simulink subsystem "MFTiresMultibodyFrontSSC"  (R2024a)
settings: Solver=VariableStepAuto  StartTime=0.0  StopTime=10.0  RelTol=1e-3
undefined symbols (not defined in the file): Alpha, AxlFL, AxlFR, AxlTrq, BrkPrs, Fx, Fy, Fz, Gamma, Kappa, Mx, My, Mz, Omega, PlntVehMultiBody, psidot, Re, Vx, Vy, WheelFL, WheelFR, X, Y, Z
libraries: nesl_utility x34, sm_lib x34, fl_lib x6
(part 2 of 2)

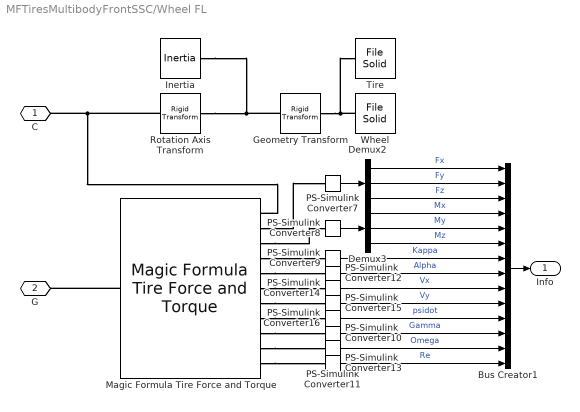
== system MFTiresMultibodyFrontSSC/Wheel FL ==
  Bus Creator1 : BusCreator  Inputs=14
  Demux2 : Demux  Outputs=3
  Demux3 : Demux  Outputs=3
  Geometry Transform : sm_lib/Frames and Transforms/Rigid Transform  RotationMethod=StandardAxis  FollAlignAxisA=+X  BaseAlignAxisA=+Y  FollAlignAxisB=+Y  BaseAlignAxisB=+Z  RotationStandardAxis=+X  RotationAngle=sideSign*180-90  RotationAngleUnits=deg  RotationArbitraryAxis=[0 0 1]  RotationSequenceAxes=FollowerAxes  RotationSequence=XYX  RotationSequenceAngles=[0 0 0]  RotationSequenceAnglesUnits=deg  RotationMatrix=[1 0 0; 0 1 0; 0 0 1]  Quaternion=[1 0 0 0]  TranslationMethod=StandardAxis  TranslationCartesianOffset=[0 0 0]  TranslationCartesianOffsetUnits=m  TranslationStandardAxis=+Y  TranslationStandardOffset=(1-2*sideSign)*0.125  TranslationStandardOffsetUnits=m  TranslationROffset=0  TranslationROffsetUnits=m  TranslationThetaOffset=0  TranslationThetaOffsetUnits=deg  TranslationZOffset=0  TranslationZOffsetUnits=m
  Inertia : sm_lib/Body Elements/Inertia  InertiaType=Custom  Mass=wheelAssm_mass  MassUnits=kg  CenterOfMass=[0 0 0]  CenterOfMassUnits=m  MomentsOfInertia=wheelAssm_I  MomentsOfInertiaUnits=kg*m^2  ProductsOfInertia=[0 0 0]  ProductsOfInertiaUnits=kg*m^2  GraphicType=None  MarkerShape=Inertia  MarkerSize=20  GraphicVisPropType=SimpleVisualProperties  GraphicDiffuseColor=[0.5 0.5 0.5]  GraphicOpacity=1.0  GraphicSpecularColor=[0.5 0.5 0.5 1.0]  GraphicAmbientColor=[0.15 0.15 0.15 1.0]  GraphicEmissiveColor=[0.0 0.0 0.0 1.0]  GraphicShininess=75
  Magic Formula Tire Force and Torque : sm_lib/Forces and Torques/Magic Formula Tire Force and Torque  TireSide=Left  TireParameters=tire_param  SlipMode=Combined  ScalingCoefficientLMUXMode=FromTireParameters  ScalingCoefficientLMUYMode=FromTireParameters  SenseContactSignal=off  TireWrenchFrame=ContactFrame  SenseTireForce=on  SenseTireTorque=on  SensePneumaticTrail=off  SenseLongitudinalSlip=on  SenseSaturatedLongitudinalSlip=off  SenseSlipAngle=on  SenseSaturatedSlipAngle=off  SenseTurnSlip=off  SenseRelativeLongitudinalVelocity=on  SenseRelativeLateralVelocity=on  SenseLongitudinalSlipVelocity=off  SenseLateralSlipVelocity=off  SenseYawVelocity=on  SenseCamberAngle=on  SenseSaturatedCamberAngle=off  SenseCamberVelocity=off  SenseSpinVelocity=on  SenseFreeRadius=off  SenseLoadedRadius=off  SenseEffectiveRollingRadius=on  SenseLongitudinalFrictionCoefficient=off  SenseLateralFrictionCoefficient=off  SenseContactBaseRotation=off  SenseContactBaseTranslation=off  SenseContactFollowerRotation=off  SenseContactFollowerTranslation=off  NumericParameters=[0.1 0.1 0.1 0.1 0.1 1e-4 1e-4 1e-7 1e-7 1e-4 1e-4 0.1 1e-4 1e-4 1e-4 1e-4 1e-4 1e-4 1e-4 1e-4 1e-4]
  PS-Simulink Converter{7..16} (10 alike) : nesl_utility/PS-Simulink Converter  PhysicalDomain=network_engine_domain  SubClassName=ps_output  LeftPortType=input  RightPortType=output  PseudoPeriodic=off  Frequencies=[]  VectorFormat=1-D array  Unit=inherit  AffineConversion=off
  Rotation Axis Transform : sm_lib/Frames and Transforms/Rigid Transform  RotationMethod=AlignedAxes  FollAlignAxisA=+X  BaseAlignAxisA=+X  FollAlignAxisB=+Z  BaseAlignAxisB=+Y  RotationStandardAxis=-X  RotationAngle=0  RotationAngleUnits=deg  RotationArbitraryAxis=[0 0 1]  RotationSequenceAxes=FollowerAxes  RotationSequence=XYX  RotationSequenceAngles=[0 0 0]  RotationSequenceAnglesUnits=deg  RotationMatrix=[1 0 0; 0 1 0; 0 0 1]  Quaternion=[1 0 0 0]  TranslationMethod=None  TranslationCartesianOffset=[0 0 0]  TranslationCartesianOffsetUnits=m  TranslationStandardAxis=+Z  TranslationStandardOffset=0  TranslationStandardOffsetUnits=m  TranslationROffset=0  TranslationROffsetUnits=m  TranslationThetaOffset=0  TranslationThetaOffsetUnits=deg  TranslationZOffset=0  TranslationZOffsetUnits=m
  Tire : sm_lib/Body Elements/File Solid  ExtGeomFileName=sm_car_heave_roll_tire.STL  UnitType=Custom  ExtGeomFileUnits=mm  StepReaderType=HEX  ExportConvexHullGeometry=off  InertiaType=Custom  BasedOnType=Density  Density=1000  DensityUnits=kg/m^3  Mass=0  MassUnits=kg  CenterOfMass=[0 0 0]  CenterOfMassUnits=m  MomentsOfInertia=[0 0 0]  MomentsOfInertiaUnits=kg*m^2  ProductsOfInertia=[0 0 0]  ProductsOfInertiaUnits=kg*m^2  GraphicType=FromGeometry  MarkerShape=Sphere  MarkerSize=10  GraphicVisPropType=SimpleVisualProperties  GraphicDiffuseColor=[0.5 0.5 0.5]  GraphicOpacity=1.0  GraphicSpecularColor=[0.5 0.5 0.5 1.0]  GraphicAmbientColor=[0.15 0.15 0.15 1.0]  GraphicEmissiveColor=[0.0 0.0 0.0 1.0]  GraphicShininess=75  DoExposeReferenceFrame=on  SerializedFrames=<Frames/>
  Wheel : sm_lib/Body Elements/File Solid  ExtGeomFileName=sm_car_heave_roll_wheel.STL  UnitType=Custom  ExtGeomFileUnits=mm  StepReaderType=HEX  ExportConvexHullGeometry=off  InertiaType=Custom  BasedOnType=Density  Density=1000  DensityUnits=kg/m^3  Mass=0  MassUnits=kg  CenterOfMass=[0 0 0]  CenterOfMassUnits=m  MomentsOfInertia=[0 0 0]  MomentsOfInertiaUnits=kg*m^2  ProductsOfInertia=[0 0 0]  ProductsOfInertiaUnits=kg*m^2  GraphicType=FromGeometry  MarkerShape=Sphere  MarkerSize=10  GraphicVisPropType=SimpleVisualProperties  GraphicDiffuseColor=[0.8 0.8 0.8]  GraphicOpacity=1.0  GraphicSpecularColor=[0.5 0.5 0.5 1.0]  GraphicAmbientColor=[0.15 0.15 0.15 1.0]  GraphicEmissiveColor=[0.0 0.0 0.0 1.0]  GraphicShininess=75  DoExposeReferenceFrame=on  SerializedFrames=<Frames/>
  C : PMIOPort  Side=Left
  G : PMIOPort  Port=2  Side=Right
  Info : Outport
  wires:
  Bus Creator1/1 -> Info/1
  Demux3/1 -> Bus Creator1/4  "Mx"
  PS-Simulink Converter12/1 -> Bus Creator1/8  "Alpha"
  PS-Simulink Converter10/1 -> Bus Creator1/12  "Gamma"
  Demux3/2 -> Bus Creator1/5  "My"
  PS-Simulink Converter8/1 -> Demux3/1
  Demux3/3 -> Bus Creator1/6  "Mz"
  Demux2/3 -> Bus Creator1/3  "Fz"
  PS-Simulink Converter16/1 -> Bus Creator1/11  "psidot"
  PS-Simulink Converter9/1 -> Bus Creator1/7  "Kappa"
  Demux2/2 -> Bus Creator1/2  "Fy"
  PS-Simulink Converter11/1 -> Bus Creator1/13  "Omega"
  PS-Simulink Converter15/1 -> Bus Creator1/10  "Vy"
  PS-Simulink Converter7/1 -> Demux2/1
  Demux2/1 -> Bus Creator1/1  "Fx"
  PS-Simulink Converter14/1 -> Bus Creator1/9  "Vx"
  PS-Simulink Converter13/1 -> Bus Creator1/14  "Re"
  connections:
  Magic Formula Tire Force and Torque/RConn3 -- PS-Simulink Converter8/LConn1
  Magic Formula Tire Force and Torque/RConn11 -- PS-Simulink Converter13/LConn1
  Magic Formula Tire Force and Torque/RConn7 -- PS-Simulink Converter15/LConn1
  Magic Formula Tire Force and Torque/RConn4 -- PS-Simulink Converter9/LConn1
  Magic Formula Tire Force and Torque/LConn1 -- G/RConn1
  Magic Formula Tire Force and Torque/RConn10 -- PS-Simulink Converter11/LConn1
  Magic Formula Tire Force and Torque/RConn8 -- PS-Simulink Converter16/LConn1
  Magic Formula Tire Force and Torque/RConn2 -- PS-Simulink Converter7/LConn1
  Magic Formula Tire Force and Torque/RConn5 -- PS-Simulink Converter12/LConn1
  Magic Formula Tire Force and Torque/RConn6 -- PS-Simulink Converter14/LConn1
  Magic Formula Tire Force and Torque/RConn9 -- PS-Simulink Converter10/LConn1
  Wheel/RConn1 -- Geometry Transform/RConn1 -- Tire/RConn1
  Inertia/RConn1 -- Geometry Transform/LConn1 -- Rotation Axis Transform/LConn1
  Magic Formula Tire Force and Torque/RConn1 -- Rotation Axis Transform/RConn1 -- C/RConn1

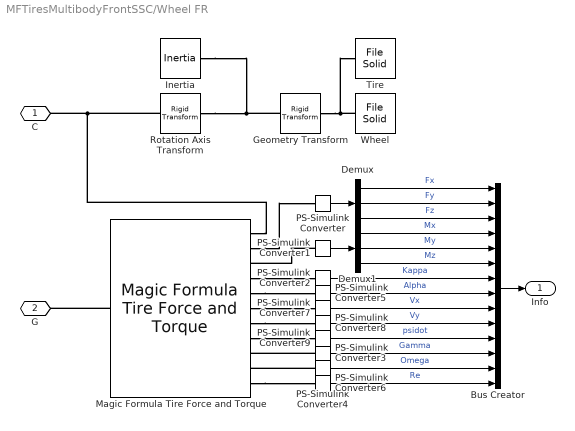
== system MFTiresMultibodyFrontSSC/Wheel FR ==
  Bus Creator : BusCreator  Inputs=14
  Demux : Demux  Outputs=3
  Demux1 : Demux  Outputs=3
  Geometry Transform : sm_lib/Frames and Transforms/Rigid Transform  RotationMethod=StandardAxis  FollAlignAxisA=+X  BaseAlignAxisA=+Y  FollAlignAxisB=+Y  BaseAlignAxisB=+Z  RotationStandardAxis=+X  RotationAngle=sideSign*180-90  RotationAngleUnits=deg  RotationArbitraryAxis=[0 0 1]  RotationSequenceAxes=FollowerAxes  RotationSequence=XYX  RotationSequenceAngles=[0 0 0]  RotationSequenceAnglesUnits=deg  RotationMatrix=[1 0 0; 0 1 0; 0 0 1]  Quaternion=[1 0 0 0]  TranslationMethod=StandardAxis  TranslationCartesianOffset=[0 0 0]  TranslationCartesianOffsetUnits=m  TranslationStandardAxis=+Y  TranslationStandardOffset=(1-2*sideSign)*0.125  TranslationStandardOffsetUnits=m  TranslationROffset=0  TranslationROffsetUnits=m  TranslationThetaOffset=0  TranslationThetaOffsetUnits=deg  TranslationZOffset=0  TranslationZOffsetUnits=m
  Inertia : sm_lib/Body Elements/Inertia  InertiaType=Custom  Mass=wheelAssm_mass  MassUnits=kg  CenterOfMass=[0 0 0]  CenterOfMassUnits=m  MomentsOfInertia=wheelAssm_I  MomentsOfInertiaUnits=kg*m^2  ProductsOfInertia=[0 0 0]  ProductsOfInertiaUnits=kg*m^2  GraphicType=None  MarkerShape=Inertia  MarkerSize=20  GraphicVisPropType=SimpleVisualProperties  GraphicDiffuseColor=[0.5 0.5 0.5]  GraphicOpacity=1.0  GraphicSpecularColor=[0.5 0.5 0.5 1.0]  GraphicAmbientColor=[0.15 0.15 0.15 1.0]  GraphicEmissiveColor=[0.0 0.0 0.0 1.0]  GraphicShininess=75
  Magic Formula Tire Force and Torque : sm_lib/Forces and Torques/Magic Formula Tire Force and Torque  TireSide=Right  TireParameters=tire_param  SlipMode=Combined  ScalingCoefficientLMUXMode=FromTireParameters  ScalingCoefficientLMUYMode=FromTireParameters  SenseContactSignal=off  TireWrenchFrame=ContactFrame  SenseTireForce=on  SenseTireTorque=on  SensePneumaticTrail=off  SenseLongitudinalSlip=on  SenseSaturatedLongitudinalSlip=off  SenseSlipAngle=on  SenseSaturatedSlipAngle=off  SenseTurnSlip=off  SenseRelativeLongitudinalVelocity=on  SenseRelativeLateralVelocity=on  SenseLongitudinalSlipVelocity=off  SenseLateralSlipVelocity=off  SenseYawVelocity=on  SenseCamberAngle=on  SenseSaturatedCamberAngle=off  SenseCamberVelocity=off  SenseSpinVelocity=on  SenseFreeRadius=off  SenseLoadedRadius=off  SenseEffectiveRollingRadius=on  SenseLongitudinalFrictionCoefficient=off  SenseLateralFrictionCoefficient=off  SenseContactBaseRotation=off  SenseContactBaseTranslation=off  SenseContactFollowerRotation=off  SenseContactFollowerTranslation=off  NumericParameters=[0.1 0.1 0.1 0.1 0.1 1e-4 1e-4 1e-7 1e-7 1e-4 1e-4 0.1 1e-4 1e-4 1e-4 1e-4 1e-4 1e-4 1e-4 1e-4 1e-4]
  PS-Simulink Converter{,1..9} (10 alike) : nesl_utility/PS-Simulink Converter  PhysicalDomain=network_engine_domain  SubClassName=ps_output  LeftPortType=input  RightPortType=output  PseudoPeriodic=off  Frequencies=[]  VectorFormat=1-D array  Unit=inherit  AffineConversion=off
  Rotation Axis Transform : sm_lib/Frames and Transforms/Rigid Transform  RotationMethod=AlignedAxes  FollAlignAxisA=+X  BaseAlignAxisA=+X  FollAlignAxisB=+Z  BaseAlignAxisB=+Y  RotationStandardAxis=-X  RotationAngle=0  RotationAngleUnits=deg  RotationArbitraryAxis=[0 0 1]  RotationSequenceAxes=FollowerAxes  RotationSequence=XYX  RotationSequenceAngles=[0 0 0]  RotationSequenceAnglesUnits=deg  RotationMatrix=[1 0 0; 0 1 0; 0 0 1]  Quaternion=[1 0 0 0]  TranslationMethod=None  TranslationCartesianOffset=[0 0 0]  TranslationCartesianOffsetUnits=m  TranslationStandardAxis=+Z  TranslationStandardOffset=0  TranslationStandardOffsetUnits=m  TranslationROffset=0  TranslationROffsetUnits=m  TranslationThetaOffset=0  TranslationThetaOffsetUnits=deg  TranslationZOffset=0  TranslationZOffsetUnits=m
  Tire : sm_lib/Body Elements/File Solid  ExtGeomFileName=sm_car_heave_roll_tire.STL  UnitType=Custom  ExtGeomFileUnits=mm  StepReaderType=HEX  ExportConvexHullGeometry=off  InertiaType=Custom  BasedOnType=Density  Density=1000  DensityUnits=kg/m^3  Mass=0  MassUnits=kg  CenterOfMass=[0 0 0]  CenterOfMassUnits=m  MomentsOfInertia=[0 0 0]  MomentsOfInertiaUnits=kg*m^2  ProductsOfInertia=[0 0 0]  ProductsOfInertiaUnits=kg*m^2  GraphicType=FromGeometry  MarkerShape=Sphere  MarkerSize=10  GraphicVisPropType=SimpleVisualProperties  GraphicDiffuseColor=[0.5 0.5 0.5]  GraphicOpacity=1.0  GraphicSpecularColor=[0.5 0.5 0.5 1.0]  GraphicAmbientColor=[0.15 0.15 0.15 1.0]  GraphicEmissiveColor=[0.0 0.0 0.0 1.0]  GraphicShininess=75  DoExposeReferenceFrame=on  SerializedFrames=<Frames/>
  Wheel : sm_lib/Body Elements/File Solid  ExtGeomFileName=sm_car_heave_roll_wheel.STL  UnitType=Custom  ExtGeomFileUnits=mm  StepReaderType=HEX  ExportConvexHullGeometry=off  InertiaType=Custom  BasedOnType=Density  Density=1000  DensityUnits=kg/m^3  Mass=0  MassUnits=kg  CenterOfMass=[0 0 0]  CenterOfMassUnits=m  MomentsOfInertia=[0 0 0]  MomentsOfInertiaUnits=kg*m^2  ProductsOfInertia=[0 0 0]  ProductsOfInertiaUnits=kg*m^2  GraphicType=FromGeometry  MarkerShape=Sphere  MarkerSize=10  GraphicVisPropType=SimpleVisualProperties  GraphicDiffuseColor=[0.8 0.8 0.8]  GraphicOpacity=1.0  GraphicSpecularColor=[0.5 0.5 0.5 1.0]  GraphicAmbientColor=[0.15 0.15 0.15 1.0]  GraphicEmissiveColor=[0.0 0.0 0.0 1.0]  GraphicShininess=75  DoExposeReferenceFrame=on  SerializedFrames=<Frames/>
  C : PMIOPort  Side=Left
  G : PMIOPort  Port=2  Side=Right
  Info : Outport
  wires:
  PS-Simulink Converter7/1 -> Bus Creator/9  "Vx"
  PS-Simulink Converter8/1 -> Bus Creator/10  "Vy"
  PS-Simulink Converter9/1 -> Bus Creator/11  "psidot"
  PS-Simulink Converter3/1 -> Bus Creator/12  "Gamma"
  PS-Simulink Converter5/1 -> Bus Creator/8  "Alpha"
  PS-Simulink Converter6/1 -> Bus Creator/14  "Re"
  PS-Simulink Converter4/1 -> Bus Creator/13  "Omega"
  PS-Simulink Converter2/1 -> Bus Creator/7  "Kappa"
  PS-Simulink Converter/1 -> Demux/1
  Demux/1 -> Bus Creator/1  "Fx"
  Demux/2 -> Bus Creator/2  "Fy"
  Demux/3 -> Bus Creator/3  "Fz"
  Demux1/3 -> Bus Creator/6  "Mz"
  Demux1/2 -> Bus Creator/5  "My"
  Demux1/1 -> Bus Creator/4  "Mx"
  PS-Simulink Converter1/1 -> Demux1/1
  Bus Creator/1 -> Info/1
  connections:
  Magic Formula Tire Force and Torque/RConn8 -- PS-Simulink Converter9/LConn1
  Magic Formula Tire Force and Torque/RConn7 -- PS-Simulink Converter8/LConn1
  Magic Formula Tire Force and Torque/RConn6 -- PS-Simulink Converter7/LConn1
  Magic Formula Tire Force and Torque/RConn11 -- PS-Simulink Converter6/LConn1
  Magic Formula Tire Force and Torque/RConn5 -- PS-Simulink Converter5/LConn1
  PS-Simulink Converter4/LConn1 -- Magic Formula Tire Force and Torque/RConn10
  PS-Simulink Converter3/LConn1 -- Magic Formula Tire Force and Torque/RConn9
  Magic Formula Tire Force and Torque/RConn4 -- PS-Simulink Converter2/LConn1
  Wheel/RConn1 -- Geometry Transform/RConn1 -- Tire/RConn1
  Inertia/RConn1 -- Geometry Transform/LConn1 -- Rotation Axis Transform/LConn1
  Magic Formula Tire Force and Torque/LConn1 -- G/RConn1
  Magic Formula Tire Force and Torque/RConn2 -- PS-Simulink Converter/LConn1
  PS-Simulink Converter1/LConn1 -- Magic Formula Tire Force and Torque/RConn3
  Rotation Axis Transform/RConn1 -- Magic Formula Tire Force and Torque/RConn1 -- C/RConn1

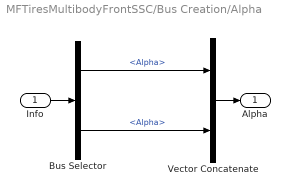
== system MFTiresMultibodyFrontSSC/Bus Creation/Alpha ==
  Info : Inport
  Bus Selector : BusSelector  OutputSignals=L.Alpha,R.Alpha
  Vector Concatenate : Concatenate
  Alpha : Outport  VectorParamsAs1DForOutWhenUnconnected=off
  wires:
  Vector Concatenate/1 -> Alpha/1
  Info/1 -> Bus Selector/1
  Bus Selector/2 -> Vector Concatenate/2  "<Alpha>"
  Bus Selector/1 -> Vector Concatenate/1  "<Alpha>"

== system MFTiresMultibodyFrontSSC/Bus Creation/BrkPrs1 ==
  In1 : Inport
  BrkPrs : Outport  VectorParamsAs1DForOutWhenUnconnected=off
  wires:
  In1/1 -> BrkPrs/1  "BrkPrs"

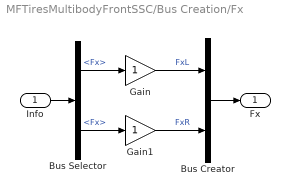
== system MFTiresMultibodyFrontSSC/Bus Creation/Fx ==
  Info : Inport
  Bus Creator : BusCreator  Inputs=2
  Bus Selector : BusSelector  OutputSignals=L.Fx,R.Fx
  Gain : Gain
  Gain1 : Gain
  Fx : Outport  VectorParamsAs1DForOutWhenUnconnected=off
  wires:
  Info/1 -> Bus Selector/1
  Bus Creator/1 -> Fx/1
  Gain1/1 -> Bus Creator/2  "FxR"
  Gain/1 -> Bus Creator/1  "FxL"
  Bus Selector/1 -> Gain/1  "<Fx>"
  Bus Selector/2 -> Gain1/1  "<Fx>"

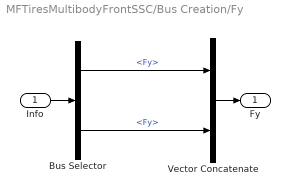
== system MFTiresMultibodyFrontSSC/Bus Creation/Fy ==
  Info : Inport
  Bus Selector : BusSelector  OutputSignals=L.Fy,R.Fy
  Vector Concatenate : Concatenate
  Fy : Outport  VectorParamsAs1DForOutWhenUnconnected=off
  wires:
  Bus Selector/2 -> Vector Concatenate/2  "<Fy>"
  Bus Selector/1 -> Vector Concatenate/1  "<Fy>"
  Vector Concatenate/1 -> Fy/1
  Info/1 -> Bus Selector/1

== system MFTiresMultibodyFrontSSC/Bus Creation/Fz ==
  Info : Inport
  Bus Selector : BusSelector  OutputSignals=L.Fz,R.Fz
  Vector Concatenate : Concatenate
  Fz : Outport  VectorParamsAs1DForOutWhenUnconnected=off
  wires:
  Bus Selector/2 -> Vector Concatenate/2  "<Fz>"
  Bus Selector/1 -> Vector Concatenate/1  "<Fz>"
  Vector Concatenate/1 -> Fz/1
  Info/1 -> Bus Selector/1

== system MFTiresMultibodyFrontSSC/Bus Creation/Gamma ==
  Info : Inport
  Bus Selector : BusSelector  OutputSignals=L.Gamma,R.Gamma
  Vector Concatenate : Concatenate
  Gamma : Outport  VectorParamsAs1DForOutWhenUnconnected=off
  wires:
  Bus Selector/1 -> Vector Concatenate/1  "<Gamma>"
  Bus Selector/2 -> Vector Concatenate/2  "<Gamma>"
  Info/1 -> Bus Selector/1
  Vector Concatenate/1 -> Gamma/1

== system MFTiresMultibodyFrontSSC/Bus Creation/Kappa ==
  Info : Inport
  Bus Selector : BusSelector  OutputSignals=L.Kappa,R.Kappa
  Vector Concatenate : Concatenate
  Kappa : Outport  VectorParamsAs1DForOutWhenUnconnected=off
  wires:
  Vector Concatenate/1 -> Kappa/1
  Info/1 -> Bus Selector/1
  Bus Selector/2 -> Vector Concatenate/2  "<Kappa>"
  Bus Selector/1 -> Vector Concatenate/1  "<Kappa>"

== system MFTiresMultibodyFrontSSC/Bus Creation/Mx ==
  Info : Inport
  Bus Selector : BusSelector  OutputSignals=L.Mx,R.Mx
  Vector Concatenate : Concatenate
  Mx : Outport  VectorParamsAs1DForOutWhenUnconnected=off
  wires:
  Bus Selector/2 -> Vector Concatenate/2  "<Mx>"
  Bus Selector/1 -> Vector Concatenate/1  "<Mx>"
  Vector Concatenate/1 -> Mx/1
  Info/1 -> Bus Selector/1

== system MFTiresMultibodyFrontSSC/Bus Creation/My ==
  Info : Inport
  Bus Selector : BusSelector  OutputSignals=L.My,R.My
  Vector Concatenate : Concatenate
  My : Outport  VectorParamsAs1DForOutWhenUnconnected=off
  wires:
  Bus Selector/2 -> Vector Concatenate/2  "<My>"
  Bus Selector/1 -> Vector Concatenate/1  "<My>"
  Vector Concatenate/1 -> My/1
  Info/1 -> Bus Selector/1

== system MFTiresMultibodyFrontSSC/Bus Creation/Mz ==
  Info : Inport
  Bus Selector : BusSelector  OutputSignals=L.Mz,R.Mz
  Vector Concatenate : Concatenate
  Mz : Outport  VectorParamsAs1DForOutWhenUnconnected=off
  wires:
  Bus Selector/2 -> Vector Concatenate/2  "<Mz>"
  Bus Selector/1 -> Vector Concatenate/1  "<Mz>"
  Vector Concatenate/1 -> Mz/1
  Info/1 -> Bus Selector/1

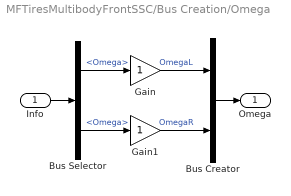
== system MFTiresMultibodyFrontSSC/Bus Creation/Omega ==
  Info : Inport
  Bus Creator : BusCreator  Inputs=2
  Bus Selector : BusSelector  OutputSignals=L.Omega,R.Omega
  Gain : Gain
  Gain1 : Gain
  Omega : Outport  VectorParamsAs1DForOutWhenUnconnected=off
  wires:
  Bus Selector/2 -> Gain1/1  "<Omega>"
  Bus Creator/1 -> Omega/1
  Info/1 -> Bus Selector/1
  Bus Selector/1 -> Gain/1  "<Omega>"
  Gain/1 -> Bus Creator/1  "OmegaL"
  Gain1/1 -> Bus Creator/2  "OmegaR"

== system MFTiresMultibodyFrontSSC/Bus Creation/Re ==
  Info : Inport
  Bus Selector : BusSelector  OutputSignals=L.Re,R.Re
  Vector Concatenate : Concatenate
  Re : Outport  VectorParamsAs1DForOutWhenUnconnected=off
  wires:
  Vector Concatenate/1 -> Re/1
  Info/1 -> Bus Selector/1
  Bus Selector/2 -> Vector Concatenate/2  "<Re>"
  Bus Selector/1 -> Vector Concatenate/1  "<Re>"

== system MFTiresMultibodyFrontSSC/Bus Creation/Vx ==
  Info : Inport
  Bus Selector : BusSelector  OutputSignals=L.Vx,R.Vx
  Vector Concatenate : Concatenate
  Vx : Outport  VectorParamsAs1DForOutWhenUnconnected=off
  wires:
  Bus Selector/1 -> Vector Concatenate/1  "<Vx>"
  Bus Selector/2 -> Vector Concatenate/2  "<Vx>"
  Info/1 -> Bus Selector/1
  Vector Concatenate/1 -> Vx/1

== system MFTiresMultibodyFrontSSC/Bus Creation/Vy ==
  Info : Inport
  Bus Selector : BusSelector  OutputSignals=L.Vy,R.Vy
  Vector Concatenate : Concatenate
  Vy : Outport  VectorParamsAs1DForOutWhenUnconnected=off
  wires:
  Vector Concatenate/1 -> Vy/1
  Info/1 -> Bus Selector/1
  Bus Selector/2 -> Vector Concatenate/2  "<Vy>"
  Bus Selector/1 -> Vector Concatenate/1  "<Vy>"

== system MFTiresMultibodyFrontSSC/Bus Creation/psidot ==
  Info : Inport
  Bus Selector : BusSelector  OutputSignals=L.psidot,R.psidot
  Vector Concatenate : Concatenate
  psidot : Outport  VectorParamsAs1DForOutWhenUnconnected=off
  wires:
  Bus Selector/1 -> Vector Concatenate/1  "<psidot>"
  Vector Concatenate/1 -> psidot/1
  Info/1 -> Bus Selector/1
  Bus Selector/2 -> Vector Concatenate/2  "<psidot>"
